simulink model "pv_array"  (R2021a)
settings: Solver=VariableStepAuto  StartTime=0.0  StopTime=10.0  RelTol=1e-3
libraries: spsPVArrayLib x1, spsVoltageMeasurementLib x1, spspowerguiLib x1
settings Model: Creator=Vaneebun  LastModifiedBy=Vaneebun

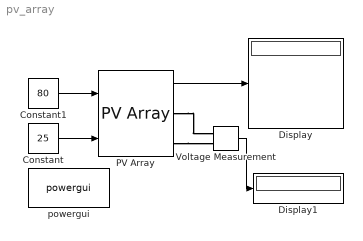
== system pv_array ==
  Constant : Constant  Value=25
  Constant1 : Constant  Value=80
  Display : Display
  Display1 : Display
  PV Array : spsPVArrayLib/PV Array  Npar=40  Nser=10  PlotType=array @ 1000 W/m2 & specified temperatures  S_vec="[ 1000  500  100 ]"  Temp_C_vec="[ 45 25  ]"  ModuleName=User-defined  PlotWhenSelected=off  Pm=200  Ncell=72  Voc=47.8  Isc=5.4  Vm=40  Im=5  beta_Voc_pc=-0.2984  alpha_Isc_pc=0.046093  beta_Voc=-0.14264  alpha_Isc=0.002489  IL=5.4099  I0=1.6974e-11  nI=0.97696  Rsh=235.9526  Rs=0.43428  RobustModel=off  RobustCellTemperature=313.3991  BAL=off  Tc=1e-6  Tfilter=5e-5
  Voltage Measurement : spsVoltageMeasurementLib/Voltage Measurement  PhasorSimulation=off  OutputType=Complex  PSBequivalent=0
  powergui : spspowerguiLib/powergui  Priority=1  SimulationMode=Discrete  SampleTime=1e-08  frequency=60  Iterations=50  frequencyindice=0  Pbase=100e6  ErrMax=1e-4  UnitsV=kV  UnitsW=MW  buscounter=0  FunctionMessages=off  echomessages=off  EnableUseOfTLC=off  CurrentSourceSwitches=off  DisableSnubberDevices=off  DisableRonSwitches=off  DisableVfSwitches=off  DisplayEquations=off  AutomaticDiscreteSolvers=off  SolverType=Tustin/Backward Euler (TBE)  Interpol=off  ExternalGateDelay=off  methode=off  Ts=100  x0status=blocks  SPID=on  SwTol=0  HookPort=off  NonlinearTolerance=1e-4  nMaxIteration=100  ContinueOnMaxIteration=off  RestoreLinks=warning  ResistiveCurrentMeasurement=off  Frange=[0:2:500]  Ylog=off  Xlog=on  ShowGrid=off  save=off  variable=ZData  structure=0  ZoomFFT=off  StartTime=0.0  cycles=1  DisplayStyle=1  fundamental=60  FreqAxis=off  MaxFrequency=1000  frequencyindicesteady=1  RmsSteady=1  display=off
  wires:
  Constant1/1 -> PV Array/1
  Constant/1 -> PV Array/2
  PV Array/1 -> Display/1
  Voltage Measurement/1 -> Display1/1
  connections:
  PV Array/RConn1 -- Voltage Measurement/LConn1
  PV Array/RConn2 -- Voltage Measurement/LConn2
